simulink model "ABS"  (R2024a)
settings: Solver=FixedStepAuto  StartTime=0.0  StopTime=10.0  RelTol=1e-3
settings Model: Creator=yuzehong  LastModifiedBy=yuzehong
settings OptimizationCC: DefaultParameterBehavior=Inlined  UseDivisionForNetSlopeComputation=on  GainParamInheritBuiltInType=on  UseFloatMulNetSlope=on  InlineInvariantSignals=on  PassReuseOutputArgsAs=Individual arguments  NoFixptDivByZeroProtection=on  EfficientFloat2IntCast=on  LifeSpan=1  OptimizeBlockOrder=speed  DifferentSizesBufferReuse=on  EfficientTunableParamExpr=on
settings DebuggingCC: ParameterTunabilityLossMsg=error
settings HardwareCC: ProdLongLongMode=on
settings SFSimCC: MATLABDynamicMemAlloc=off
settings RTWCC: Description=Embedded Coder  SystemTargetFile=ert.tlc  TemplateMakefile=ert_default_tmf
settings CodeAppCC: GenerateComments=off  IgnoreCustomStorageClasses=off  OperatorAnnotations=on  SimulinkDataObjDesc=on  SFDataObjDesc=on  CustomSymbolStrGlobalVar=rt$N$M  CustomSymbolStrType=$N$M  CustomSymbolStrFcn=$N$M$F  CustomSymbolStrMacro=$N$M  SimulinkBlockComments=off
settings ERTTargetCC: TargetLangStandard=C99 (ISO)  GenerateSampleERTMain=on  IncludeMdlTerminateFcn=off  CombineSignalStateStructs=on  SupportAbsoluteTime=off  CodeInterfacePackaging=Reusable function  SupportComplex=off  SupportContinuousTime=on  InlinedParameterPlacement=NonHierarchical  ERTCustomFileTemplate=example_file_process.tlc  ERTFilePackagingFormat=CompactWithDataFile

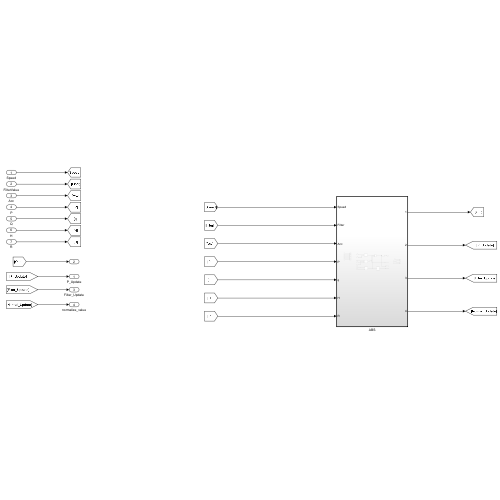
[thumbnail: Simulink's stored preview of the top-level diagram]
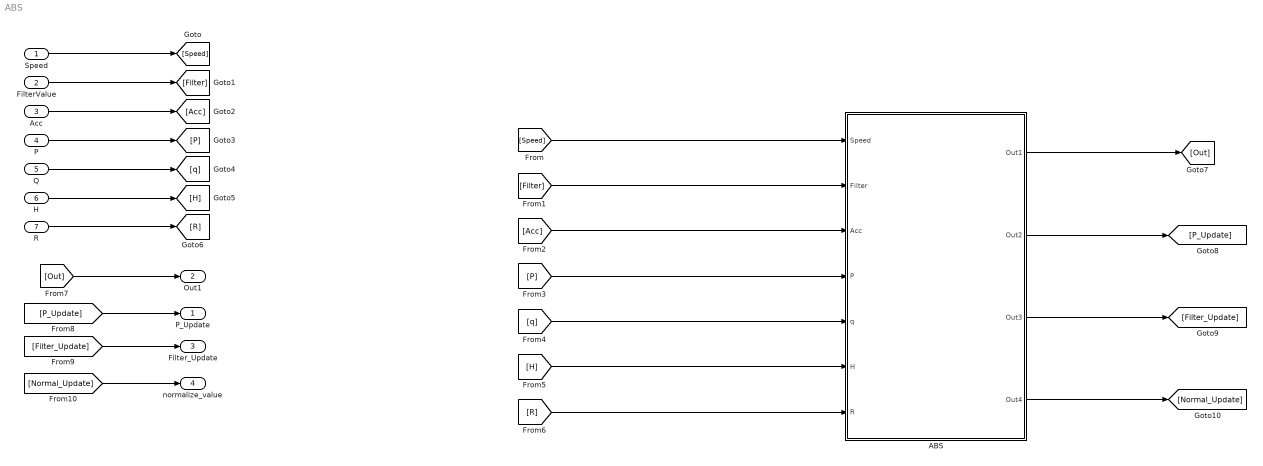
== system ABS ==
  Speed : Inport  OutDataTypeStr=int32  PortDimensions=32
  FilterValue : Inport  Port=2  OutDataTypeStr=int32  PortDimensions=32
  Acc : Inport  Port=3  OutDataTypeStr=int16  PortDimensions=32
  P : Inport  Port=4  OutDataTypeStr=int16  PortDimensions=32
  Q : Inport  Port=5  OutDataTypeStr=int32  PortDimensions=32
  H : Inport  Port=6  OutDataTypeStr=int32  PortDimensions=32
  R : Inport  Port=7  OutDataTypeStr=int32  PortDimensions=32
  ABS : Subsystem  TreatAsAtomicUnit=on
  P_Update : Outport
  Out1 : Outport  Port=2  OutDataTypeStr=int32  PortDimensions=32
  Filter_Update : Outport  Port=3  OutDataTypeStr=int32  PortDimensions=32
  normalize_value : Outport  Port=4  OutDataTypeStr=single  PortDimensions=32
  wires:
  Speed/1 -> [Speed]
  [Speed] -> ABS/1(Speed)
  FilterValue/1 -> [Filter]
  [Filter] -> ABS/2(Filter)
  Acc/1 -> [Acc]
  [Acc] -> ABS/3(Acc)
  P/1 -> [P]
  [P] -> ABS/4(P)
  Q/1 -> [q]
  [q] -> ABS/5(q)
  H/1 -> [H]
  [H] -> ABS/6(H)
  R/1 -> [R]
  [R] -> ABS/7(R)
  ABS/1(Out1) -> [Out]
  [Out] -> Out1/1
  ABS/2(Out2) -> [P_Update]
  [P_Update] -> P_Update/1
  ABS/3(Out3) -> [Filter_Update]
  [Filter_Update] -> Filter_Update/1
  ABS/4(Out4) -> [Normal_Update]
  [Normal_Update] -> normalize_value/1

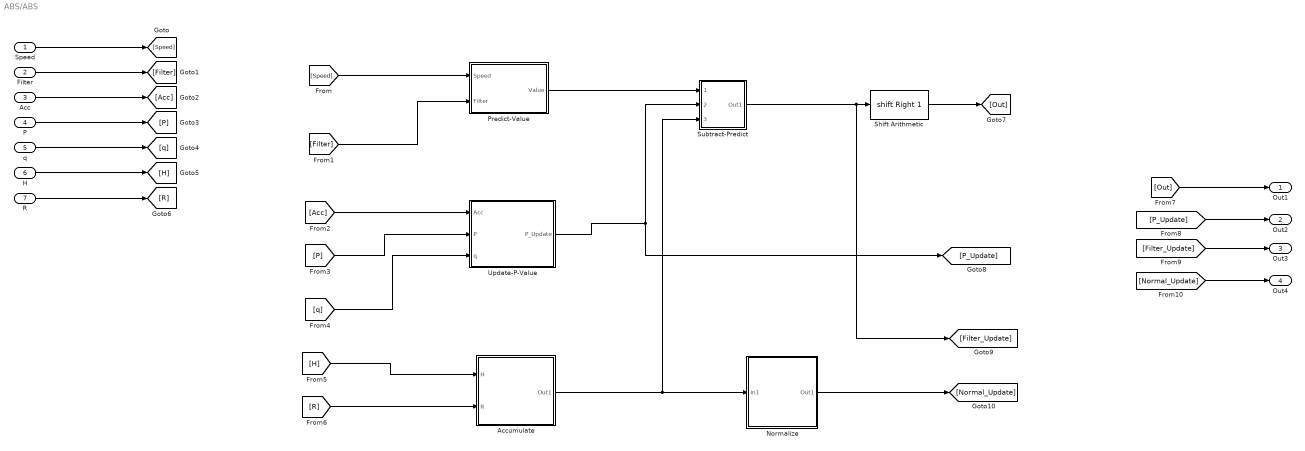
== system ABS/ABS ==
  Speed : Inport
  Filter : Inport  Port=2
  Acc : Inport  Port=3
  P : Inport  Port=4
  q : Inport  Port=5
  H : Inport  Port=6
  R : Inport  Port=7
  Accumulate : Subsystem  TreatAsAtomicUnit=on
  Normalize : Subsystem  TreatAsAtomicUnit=on
  Predict-Value : Subsystem  TreatAsAtomicUnit=on
  Shift Arithmetic : ArithShift  BitShiftNumber=1  BitShiftDirection=Right
  Subtract-Predict : Subsystem  TreatAsAtomicUnit=on
  Update-P-Value : Subsystem  TreatAsAtomicUnit=on
  Out1 : Outport
  Out2 : Outport  Port=2
  Out3 : Outport  Port=3
  Out4 : Outport  Port=4
  wires:
  q/1 -> [q]
  R/1 -> [R]
  P/1 -> [P]
  H/1 -> [H]
  Acc/1 -> [Acc]
  Speed/1 -> [Speed]
  Filter/1 -> [Filter]
  [P_Update] -> Out2/1
  [Normal_Update] -> Out4/1
  [Out] -> Out1/1
  [Filter_Update] -> Out3/1
  Shift Arithmetic/1 -> [Out]
  Normalize/1(Out1) -> [Normal_Update]
  [Speed] -> Predict-Value/1(Speed)
  [Filter] -> Predict-Value/2(Filter)
  Update-P-Value/1(P_Update) -> Subtract-Predict/2(P_Update), [P_Update]
  [Acc] -> Update-P-Value/1(Acc)
  [P] -> Update-P-Value/2(P)
  [q] -> Update-P-Value/3(q)
  Accumulate/1(Out1) -> Subtract-Predict/3(Accumulate), Normalize/1(In1)
  [H] -> Accumulate/1(H)
  [R] -> Accumulate/2(R)
  Subtract-Predict/1(Out1) -> [Filter_Update], Shift Arithmetic/1
  Predict-Value/1(Value) -> Subtract-Predict/1(Predict_Value)

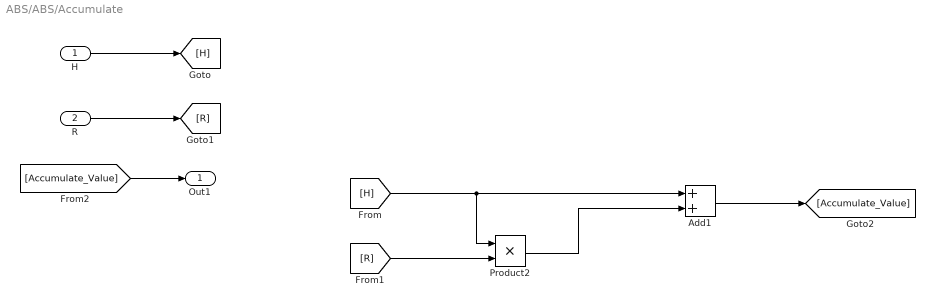
== system ABS/ABS/Accumulate ==
  H : Inport
  R : Inport  Port=2
  Add1 : Sum  OutDataTypeStr=int32  SaturateOnIntegerOverflow=on
  Product2 : Product  OutDataTypeStr=int32
  Out1 : Outport
  wires:
  Product2/1 -> Add1/2
  H/1 -> [H]
  [H] -> Product2/1, Add1/1
  R/1 -> [R]
  [R] -> Product2/2
  [Accumulate_Value] -> Out1/1
  Add1/1 -> [Accumulate_Value]

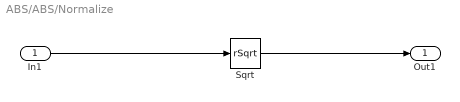
== system ABS/ABS/Normalize ==
  In1 : Inport
  Sqrt : Sqrt  Operator=rSqrt  OutDataTypeStr=single  RndMeth=Simplest  SaturateOnIntegerOverflow=off
  Out1 : Outport
  wires:
  In1/1 -> Sqrt/1
  Sqrt/1 -> Out1/1

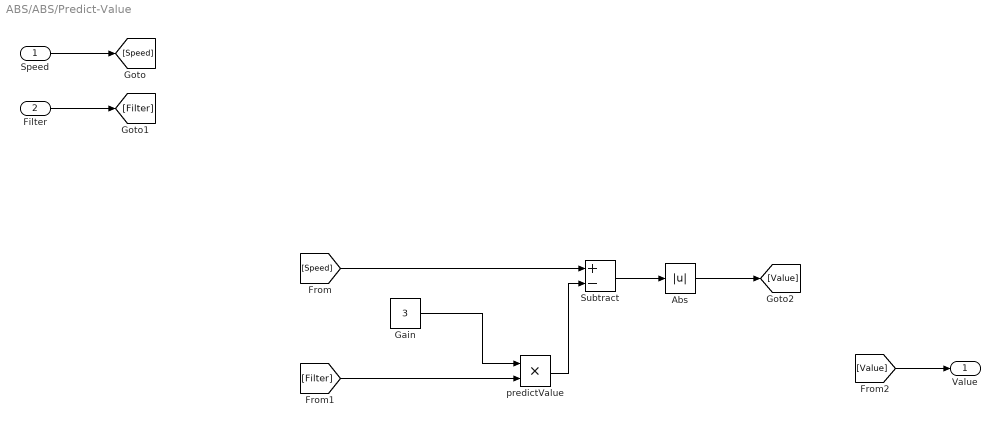
== system ABS/ABS/Predict-Value ==
  Speed : Inport
  Filter : Inport  Port=2
  Abs : Abs  SaturateOnIntegerOverflow=off
  Gain : Constant  Value=3  OutDataTypeStr=int32
  Subtract : Sum  Inputs=+-  OutDataTypeStr=int32
  predictValue : Product  OutDataTypeStr=int32
  Value : Outport
  wires:
  predictValue/1 -> Subtract/2
  Subtract/1 -> Abs/1
  Gain/1 -> predictValue/1
  Speed/1 -> [Speed]
  [Speed] -> Subtract/1
  Filter/1 -> [Filter]
  [Filter] -> predictValue/2
  [Value] -> Value/1
  Abs/1 -> [Value]

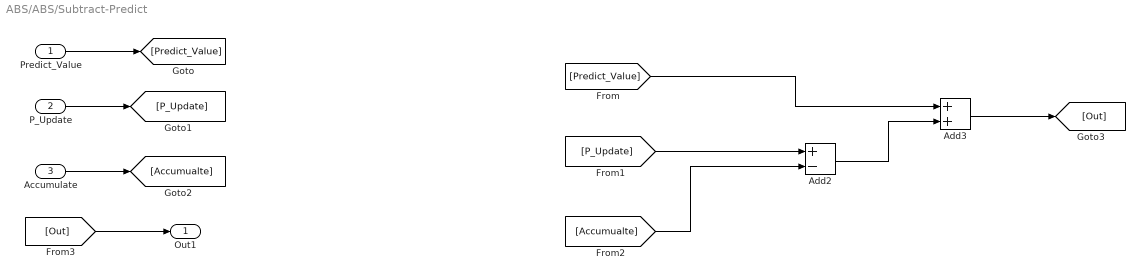
== system ABS/ABS/Subtract-Predict ==
  Predict_Value : Inport
  P_Update : Inport  Port=2
  Accumulate : Inport  Port=3
  Add2 : Sum  Inputs=+-  OutDataTypeStr=int32  SaturateOnIntegerOverflow=on
  Add3 : Sum  OutDataTypeStr=int32  SaturateOnIntegerOverflow=on
  Out1 : Outport
  wires:
  Add2/1 -> Add3/2
  Predict_Value/1 -> [Predict_Value]
  [Predict_Value] -> Add3/1
  P_Update/1 -> [P_Update]
  [P_Update] -> Add2/1
  Accumulate/1 -> [Accumualte]
  [Accumualte] -> Add2/2
  [Out] -> Out1/1
  Add3/1 -> [Out]

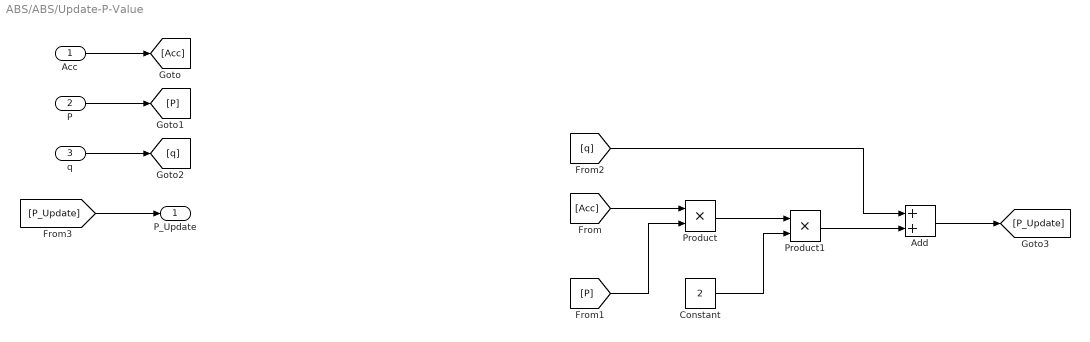
== system ABS/ABS/Update-P-Value ==
  Acc : Inport
  P : Inport  Port=2
  q : Inport  Port=3
  Add : Sum  OutDataTypeStr=int32  SaturateOnIntegerOverflow=on
  Constant : Constant  Value=2  OutDataTypeStr=int32
  Product : Product  OutDataTypeStr=int32
  Product1 : Product  OutDataTypeStr=int32  SaturateOnIntegerOverflow=on
  P_Update : Outport
  wires:
  Product1/1 -> Add/2
  Constant/1 -> Product1/2
  Product/1 -> Product1/1
  Acc/1 -> [Acc]
  [Acc] -> Product/1
  P/1 -> [P]
  [P] -> Product/2
  q/1 -> [q]
  [q] -> Add/1
  [P_Update] -> P_Update/1
  Add/1 -> [P_Update]
